simulink model "RoboticFish_NGC"  (R2023b)
settings: Solver=ode4  StartTime=0.0  StopTime=89  FixedStep=0.00025  RelTol=1e-3  EnableMultiTasking=on
undefined symbols (not defined in the file): Ref, uCMD
libraries: sharedutil x11, slpidlib x8, dspsigops x2, matrix_library x1, SignalEditorBlockLib x1, vrlib x1
(part 1 of 3)
settings Model: Creator=Waqas Ali Waqar  LastModifiedBy=Dimau
settings SolverCC: ConcurrentTasks=on  AlgebraicLoopSolver=TrustRegion  AutoInsertRateTranBlk=on  InsertRTBMode=Never (minimum delay)
settings DataIOCC: SaveFormat=StructureWithTime
settings OptimizationCC: BlockReduction=off  OptimizeBlockIOStorage=off  BufferReuse=off  GlobalBufferReuse=off  ExpressionFolding=off  PassReuseOutputArgsThreshold=0  LocalBlockOutputs=off  OptimizeBlockOrder=speed  OptimizeDataStoreBuffers=off  BusAssignmentInplaceUpdate=off
settings DebuggingCC: ParameterTunabilityLossMsg=error  UnconnectedInputMsg=warning  UnconnectedOutputMsg=warning  UnconnectedLineMsg=warning
settings HardwareCC: ProdBitPerPointer=32  ProdBitPerSizeT=32  ProdBitPerPtrDiffT=32  ProdLargestAtomicFloat=None  ProdWordSize=32  ProdLongLongMode=on  ProdHWDeviceType=Generic->32-bit x86 compatible
settings ModelReferenceCC: EnableRefExpFcnMdlSchedulingChecks=on
settings SFSimCC: MATLABDynamicMemAlloc=off  CustomCodeUndefinedFunction=UseInterfaceOnly
settings RTWCC: GenerateReport=on  RTWVerbose=off  LaunchReport=on  RTWCompilerOptimization=on  DLArmComputeVersion=19.05
settings CodeAppCC: ForceParamTrailComments=on  OperatorAnnotations=on
settings GRTTargetCC: TargetLangStandard=C89/C90 (ANSI)

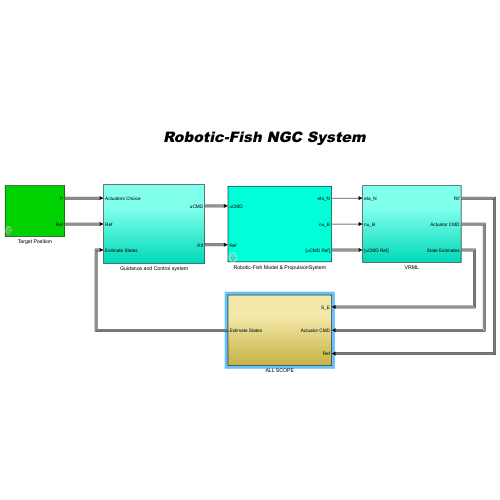
[thumbnail: Simulink's stored preview of the top-level diagram]
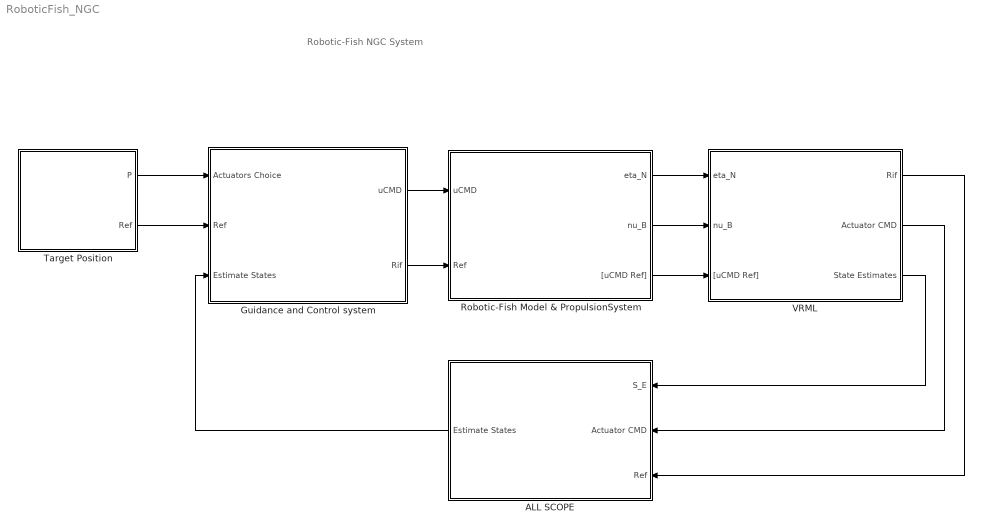
== system RoboticFish_NGC ==
  note: Robotic-Fish NGC System
  ALL SCOPE : Subsystem
  Guidance and Control system : Subsystem
  Robotic-Fish Model & PropulsionSystem : Subsystem  mask{Ig=[0.0198 0 0;0 0.9266 0;0 0 0.9266], m=11.3, rho=1000, R=0.06, L=1, cdf=0.5, cdt=1, W=107.91, B=107.91, rG_B=[0;0;0], rB_B=[0;0;0], DL=diag([0;0;0;0;0;0]), Kt0=1.16, Km1=0.5, Kt1=0.5, Km2=0.073, Kt2=1.26, beta=-4.95, Kl1=0.5, sigma=-3.52, Kl2=5.16, epsilon=-3.51, c=0.1, S=0, a0=0, a2=0, a1=0, Theta0deg=23, cL=2, xfin=0.11, yfin=0.11, zfin=0.75, Max_Delta=45, Min_Delta=-45, Sfin=0.017, HT1Max=1.12, e1=[1;0;0], r1=[0;-0.11;0], HT2Max=1.12, e2=[1;0;0], r2=[0;0.11;0], VT1Max=1.12, e3=[0;0;1], r3=[0;0;-0.03]}
      mask prompts: Ig "Inertia Tensor Ig (Kg*m^2)"; m "Mass m (Kg)"; rho "Seawater Density rho (Kg/m)"; R "Body Radius R (m)"; L "Body Lenght L (m)"; cdf "Drag Weight cdf"; cdt "Drag Weight cdt [0.8-1.2]"; W "Weight (N)"; B "Buoyancy (N)"; rG_B "rG_B (m)"; rB_B "rB_B (m)"; DL "Linear Damping Matrix"; c "c-Foil Mean Chord (m)"; S "S-Foil area (m^2)"; a0 "a0 (Kg*m^2)"; a2 "a2 (Kg*m^2)"; a1 "a1 (Kg*m^2)"; Theta0deg "Theta0-Oscillation amplitude (deg)"; cL "fin lift coefficient  cL"; xfin "fin axial position xfin (m)"; yfin "fin axial position yfin (m)"; zfin "fin axial position zfin (m)"; Max_Delta "Max fin rotation angle (deg)"; Min_Delta "Min fin rotation angle (deg)"; Sfin "fin platform area Sfin (m^2)"; HT1Max "Max Thrust (HT1):"; e1 "e1 (HT1):"; r1 "r1 (HT1):"; HT2Max "Max Thrust (HT2):"; e2 "e2 (HT2 ):"; r2 "r2 (HT2):"; VT1Max "Max Thrust (VT1):"; e3 "e3 (VT1):"; r3 "r3 (VT1):"
      mask init:
      | %%%%%%%%%%%%%%%%%%%%%%%%%%%%%%%%%%%%%%%%%%%%%%%%%%%%%%%
      | %%%%%%%%%%%%%%%%%%%  DINAMICA  %%%%%%%%%%%%%%%%%%%%%%%%
      | %%%%%%%%%%%%%%%%%%%%%%%%%%%%%%%%%%%%%%%%%%%%%%%%%%%%%%%
      | 
      | % Matrice di inerzia del corpo rigido
      | Ib = Ig-m*skewsymm(rG_B)*skewsymm(rG_B);
      | MRB = [m*eye(3,3) -m*skewsymm(rG_B); m*skewsymm(rG_B) Ib];
      | 
      | %Masse aggiunte
      | X_udot = 0.1*m;
      | Y_vdot = pi*rho*R^2*L;
      | Z_wdot = pi*rho*R^2*L;
      | K_pdot = 0;
      | M_qdot = (pi*rho*R^2*L^3)/12;
      | N_rdot = (pi*rho*R^2*L^3)/12;
      | 
      | %Matrice delle masse aggiunte
      | MA = diag([X_udot;Y_vdot;Z_wdot;K_pdot;M_qdot;N_rdot]);
      | 
      | %Matrice di inerzia (incluse le masse aggiunte)
      | M = MRB + MA;
      | inv_M = inv(M);
      | M11 = MA(1:3,1:3);    M12 = MA(1:3,4:6);
      | M21 = MA(4:6,1:3);    M22 = MA(4:6,4:6);
      | 
      | %%Attrito viscoso
      | 
      | %Aree
      | Af = pi*R^2;
      | At = 2*pi*R;
      | 
      | %Coefficienti
      | X_uu = 2*rho*Af*cdf/2;
      | Y_vv = rho*At*cdt/2;
      | Z_ww = rho*At*cdt/2;
      | K_pp = (rho*At*cdt*L^3)/16;
      | M_qq = (rho*At*cdt*L^3)/16;
      | N_rr = (rho*At*cdt*L^3)/16;
      | 
      | dQ = ([X_uu;Y_vv;Z_ww;K_pp;M_qq;N_rr]);
      | 
      | 
      | %%%%%%%%%%%%%%%%%%%%%%%%%%%%%%%%%%%%%%%%%%%%%%%%%%%%%%%
      | %%%%%%%%%%%%%%%%%%%  PROP HT3  %%%%%%%%%%%%%%%%%%%%%%%%
      | %%%%%%%%%%%%%%%%%%%%%%%%%%%%%%%%%%%%%%%%%%%%%%%%%%%%%%%
      | 
      | Theta0=Theta0deg*pi/180
      | TanTheta0=tan(Theta0)
      | 
      | %%%%%%%%%%%%%%%%%%%%%%%%%%%%%%%%%%%%%%%%%%%%%%%%%%%%%%%
      | %%%%%%%%%%%%%%%%%%%  PROP HT1 HT2 VT1  %%%%%%%%%%%%%%%%
      | %%%%%%%%%%%%%%%%%%%%%%%%%%%%%%%%%%%%%%%%%%%%%%%%%%%%%%%
      | 
      | K1 = HT1Max*9.81;
      | K2 = HT2Max*9.81;
      | K3 = VT1Max*9.81;
      | HT_prop = [e1 e2;skewsymm(r1)*e1 skewsymm(r2)*e2]*diag([K1;K2]);
      | VT_prop = [e3 ;skewsymm(r3)*e3 ]*K3;
      | 
      | 
      | %%%%%%%%%%%%%%%%%%%%%%%%%%%%%%%%%%%%%%%%%%%%%%%%%%%%%%%
      | %%%%%%%%%%%%%%%%%%%  PROP VT1 VT2  %%%%%%%%%%%%%%%%%%%%
      | %%%%%%%%%%%%%%%%%%%%%%%%%%%%%%%%%%%%%%%%%%%%%%%%%%%%%%%
      | 
      | Max_Delta_rad=Max_Delta*pi/180;
      | Min_Delta_rad=Min_Delta*pi/180;
      mask DialogControl DescGroupVar Prompt: Robotic Fish Paramteres
      mask DialogControl Container14 Prompt: Robotic Fish Parameters
      mask DialogControl Container17 Prompt: Caudal Fin Parameters
      mask DialogControl Container18 Prompt: Pectoral Fins Parameters
      mask DialogControl Container19 Prompt: Thrusters Parameters
  Target Position : Subsystem  mask{AC=Only Caudal Fin, ST=Way-Points based Path, Xr=10, Yr=0, Zr=0}
      mask init:
      | if (ST == 1)
      |     Flag=0;
      | end
      | if (ST == 2)
      |     Flag=1;
      | end
      | 
      | if (AC == 1)
      |     PropChoice=0;
      | end
      | if (AC == 2)
      |     PropChoice=1;
      | end
      | if (AC == 3)
      |     PropChoice=2;
      | end
      mask TypeOptions AC: Normal | Only Propeller | Only Caudal Fin
      mask TypeOptions ST: Way-Points based Path | Way-Point Position
      mask DialogControl DescGroupVar Prompt: Target Position
      mask DialogControl Container8 Prompt: Actuator Choice
      mask DialogControl Container7 Prompt: Select Target
      mask DialogControl Container9 Prompt: Way-Point position
  "VRML " : Subsystem
  wires:
  Robotic-Fish Model & PropulsionSystem/2(nu_B) -> "VRML "/2(nu_B)
  Target Position/1(" P") -> Guidance and Control system/1(Actuators Choice)
  Robotic-Fish Model & PropulsionSystem/1(eta_N) -> "VRML "/1(eta_N)
  Target Position/2(Ref) -> Guidance and Control system/2(Ref)
  ALL SCOPE/1(Estimate States) -> Guidance and Control system/3("Estimate States ")
  "VRML "/3(State Estimates) -> ALL SCOPE/1(S_E)
  "VRML "/2(Actuator CMD) -> ALL SCOPE/2(Actuator CMD)
  "VRML "/1(Rif) -> ALL SCOPE/3(Ref)
  Robotic-Fish Model & PropulsionSystem/3("[uCMD Ref]") -> "VRML "/3("[uCMD Ref]")
  Guidance and Control system/1(uCMD) -> Robotic-Fish Model & PropulsionSystem/1(uCMD)
  Guidance and Control system/2(Rif) -> Robotic-Fish Model & PropulsionSystem/2(Ref)

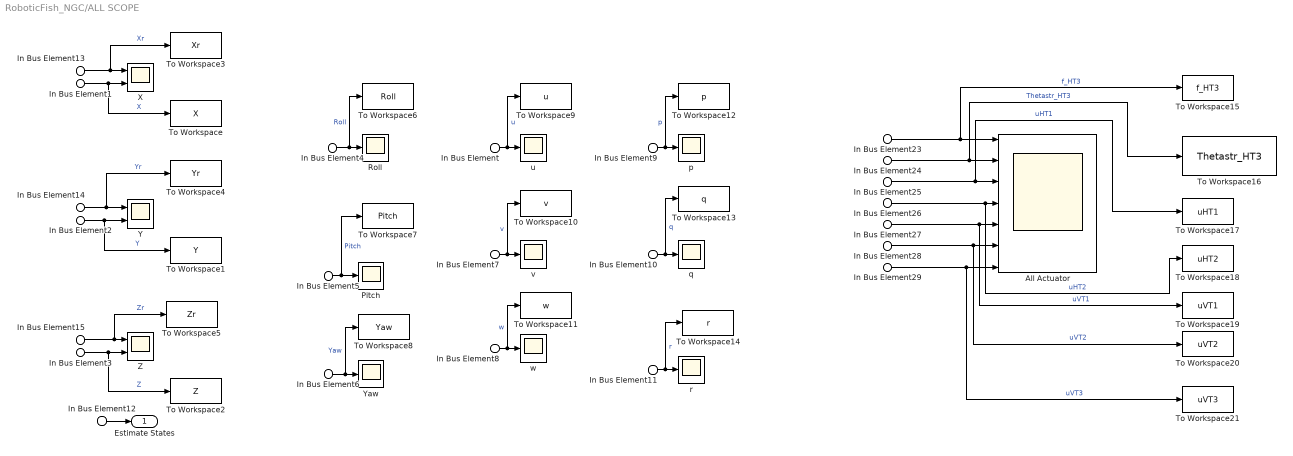
== system RoboticFish_NGC/ALL SCOPE ==
  In Bus Element12 : Inport  PortName=S_E
  In Bus Element2 : Inport  PortName=S_E  Element=Position.Y
  In Bus Element3 : Inport  PortName=S_E  Element=Position.Z
  In Bus Element4 : Inport  PortName=S_E  Element=Position.Roll
  In Bus Element5 : Inport  PortName=S_E  Element=Position.Pitch
  In Bus Element6 : Inport  PortName=S_E  Element=Position.Yaw
  In Bus Element1 : Inport  PortName=S_E  Element=Position.X
  In Bus Element : Inport  PortName=S_E  Element=Velocity.u
  In Bus Element7 : Inport  PortName=S_E  Element=Velocity.v
  In Bus Element8 : Inport  PortName=S_E  Element=Velocity.w
  In Bus Element9 : Inport  PortName=S_E  Element=Velocity.p
  In Bus Element10 : Inport  PortName=S_E  Element=Velocity.q
  In Bus Element11 : Inport  PortName=S_E  Element=Velocity.r
  In Bus Element23 : Inport  Port=2  PortName=Actuator CMD  Element=f_HT3
  In Bus Element24 : Inport  Port=2  PortName=Actuator CMD  Element=Thetastr_HT3
  In Bus Element25 : Inport  Port=2  PortName=Actuator CMD  Element=uHT1
  In Bus Element26 : Inport  Port=2  PortName=Actuator CMD  Element=uHT2
  In Bus Element27 : Inport  Port=2  PortName=Actuator CMD  Element=uVT1
  In Bus Element28 : Inport  Port=2  PortName=Actuator CMD  Element=D_VT2
  In Bus Element29 : Inport  Port=2  PortName=Actuator CMD  Element=D_VT3
  In Bus Element13 : Inport  Port=3  PortName=Ref  Element=Xr
  In Bus Element14 : Inport  Port=3  PortName=Ref  Element=Yr
  In Bus Element15 : Inport  Port=3  PortName=Ref  Element=Zr
  All Actuator : Scope  NumInputPorts=7
  Pitch : Scope
  Roll : Scope
  To Workspace : ToWorkspace  VariableName=X  SampleTime=-1
  To Workspace1 : ToWorkspace  VariableName=Y  SampleTime=-1
  To Workspace10 : ToWorkspace  VariableName=v  SampleTime=-1
  To Workspace11 : ToWorkspace  VariableName=w  SampleTime=-1
  To Workspace12 : ToWorkspace  VariableName=p  SampleTime=-1
  To Workspace13 : ToWorkspace  VariableName=q  SampleTime=-1
  To Workspace14 : ToWorkspace  VariableName=r  SampleTime=-1
  To Workspace15 : ToWorkspace  VariableName=f_HT3  SampleTime=-1
  To Workspace16 : ToWorkspace  VariableName=Thetastr_HT3  SampleTime=-1
  To Workspace17 : ToWorkspace  VariableName=uHT1  SampleTime=-1
  To Workspace18 : ToWorkspace  VariableName=uHT2  SampleTime=-1
  To Workspace19 : ToWorkspace  VariableName=uVT1  SampleTime=-1
  To Workspace2 : ToWorkspace  VariableName=Z  SampleTime=-1
  To Workspace20 : ToWorkspace  VariableName=uVT2  SampleTime=-1
  To Workspace21 : ToWorkspace  VariableName=uVT3  SampleTime=-1
  To Workspace3 : ToWorkspace  VariableName=Xr  SampleTime=-1
  To Workspace4 : ToWorkspace  VariableName=Yr  SampleTime=-1
  To Workspace5 : ToWorkspace  VariableName=Zr  SampleTime=-1
  To Workspace6 : ToWorkspace  VariableName=Roll  SampleTime=-1
  To Workspace7 : ToWorkspace  VariableName=Pitch  SampleTime=-1
  To Workspace8 : ToWorkspace  VariableName=Yaw  SampleTime=-1
  To Workspace9 : ToWorkspace  VariableName=u  SampleTime=-1
  X : Scope  NumInputPorts=2
  Y : Scope  NumInputPorts=2
  Yaw : Scope
  Z : Scope  NumInputPorts=2
  p : Scope
  q : Scope
  r : Scope
  u : Scope
  v : Scope
  w : Scope
  Estimate States : Outport  VectorParamsAs1DForOutWhenUnconnected=off
  wires:
  In Bus Element4/1 -> To Workspace6/1, Roll/1  "Roll"
  In Bus Element5/1 -> To Workspace7/1, Pitch/1  "Pitch"
  In Bus Element6/1 -> To Workspace8/1, Yaw/1  "Yaw"
  In Bus Element/1 -> To Workspace9/1, u/1  "u"
  In Bus Element7/1 -> To Workspace10/1, v/1  "v"
  In Bus Element8/1 -> To Workspace11/1, w/1  "w"
  In Bus Element9/1 -> To Workspace12/1, p/1  "p"
  In Bus Element10/1 -> To Workspace13/1, q/1  "q"
  In Bus Element11/1 -> To Workspace14/1, r/1  "r"
  In Bus Element12/1 -> Estimate States/1
  In Bus Element15/1 -> To Workspace5/1, Z/1  "Zr"
  In Bus Element3/1 -> To Workspace2/1, Z/2  "Z"
  In Bus Element2/1 -> Y/2, To Workspace1/1  "Y"
  In Bus Element14/1 -> To Workspace4/1, Y/1  "Yr"
  In Bus Element23/1 -> To Workspace15/1, All Actuator/1  "f_HT3"
  In Bus Element24/1 -> All Actuator/2, To Workspace16/1  "Thetastr_HT3"
  In Bus Element25/1 -> To Workspace17/1, All Actuator/3  "uHT1"
  In Bus Element26/1 -> To Workspace18/1, All Actuator/4  "uHT2"
  In Bus Element27/1 -> All Actuator/5, To Workspace19/1  "uVT1"
  In Bus Element28/1 -> All Actuator/6, To Workspace20/1  "uVT2"
  In Bus Element29/1 -> All Actuator/7, To Workspace21/1  "uVT3"
  In Bus Element1/1 -> X/2, To Workspace/1  "X"
  In Bus Element13/1 -> X/1, To Workspace3/1  "Xr"

== system RoboticFish_NGC/Guidance and Control system ==
  note: [X Y Z]
  note: [X Y Z] at the
      | current time
  note: [D, Yaw_d, Ze]
  note: "uCMD" vector is formed by the control signals of the robotic fish actuators
  note: Waypoints [Xr Yr Zr]
  Actuators Choice : Inport
  Ref : Inport  Port=2
  "Estimate States " : Inport  Port=3
  " Control system" : Subsystem
  " Guidance system" : Subsystem
  uCMD : Outport  VectorParamsAs1DForOutWhenUnconnected=off
  Rif : Outport  Port=2  VectorParamsAs1DForOutWhenUnconnected=off
  wires:
  "Estimate States "/1 -> " Guidance system"/2(Estimate States I)
  Ref/1 -> Rif/1, " Guidance system"/1(Ref)
  " Guidance system"/1("LOS ") -> " Control system"/1(LOS)
  Actuators Choice/1 -> " Control system"/2(Actuators Choice)
  " Guidance system"/2(Estimate States O) -> " Control system"/3(Estimate States)
  " Control system"/1(uCMD) -> uCMD/1

== system RoboticFish_NGC/Robotic-Fish Model & PropulsionSystem ==
  uCMD : Inport
  In Bus Element1 : Inport  Port=2  PortName=Ref
  Bus Creator : BusCreator  Inputs=2
  Memory : Memory
  Propulsion System : Subsystem
  RF Dynamics and Kinematics (Attitude rappresentation: Quaternions) : Subsystem
      mask Display: image('RF.png');
  eta_N : Outport  VectorParamsAs1DForOutWhenUnconnected=off
  nu_B : Outport  Port=2  VectorParamsAs1DForOutWhenUnconnected=off
  "[uCMD Ref]" : Outport  Port=3  VectorParamsAs1DForOutWhenUnconnected=off
  wires:
  RF Dynamics and Kinematics (Attitude rappresentation: Quaternions)/1(nu_B) -> nu_B/1, Memory/1  "[u    v    w    p    q    r]"
  Memory/1 -> Propulsion System/1(nu_B)
  RF Dynamics and Kinematics (Attitude rappresentation: Quaternions)/2(eta_N) -> eta_N/1  "[x   y   z  q0  q1  q2  q3]"
  uCMD/1 -> Propulsion System/2(uCMD)
  Propulsion System/2(ucmd) -> Bus Creator/1  "uCMD"
  Propulsion System/1(Tau_B) -> RF Dynamics and Kinematics (Attitude rappresentation: Quaternions)/1(tau_B)  "[Tau_X, Tau_Y, Tau_Z, Tau_Roll, Tau_Pitch, Tau_Yaw]"
  In Bus Element1/1 -> Bus Creator/2  "Ref"
  Bus Creator/1 -> "[uCMD Ref]"/1

== system RoboticFish_NGC/Target Position ==
  note: By means of a radio button, it is possible to choose how the vehicle is actuated.
      |
      | 0) “Normal” operation which involves the use of the caudal fin for surge motion, the lateral propellers for steering.
      |
      | 1) “Only Propeller” operation, where the propellers are used for both surge motion and steering.
      |
      | 2) "Only Caudal Fin" operation which involves only the use of the caudal fin for surge motion and steering.
  note: The control panel provides a radio button that allows you to choose the type of target to be reached.
      |
      | 0) “Way-Points based Path” allows you to choose Path consisting of a multiple waypoint that can be generated from the “Waypoints generator” block, which is a Simulink block that creates a group of signals (“Signal Builder”).
      |
      | 1) “Way-Point Position” consists in choosing the x y z coordinate of the reference, essentially it consists of a set-point.
  note: u1 (if u2 = 1)
  note: u3 (if u2 = 0)
  note: Waypoints [Xr Yr Zr]
  note: u2
  note: u3 Waypoints based Path
  note: u1 Waypoint Position
  Bus Creator : BusCreator  Inputs=3
  Bus Creator1 : BusCreator  Inputs=3
  Constant : Constant  Value=Flag
  Constant1 : Constant  Value=Xr
  Constant2 : Constant  Value=Yr
  Constant3 : Constant  Value=Zr
  Constant4 : Constant  Value=PropChoice
  Signal Editor : SignalEditorBlockLib/Signal Editor  FileName=waypoint_generator.mat  ActiveScenario=Scenario  ActiveSignal=Xr  IsBus=off  OutputBusObjectStr=Bus: BusObject  SampleTime=0  Interpolate=off  ZeroCross=off  OutputAfterFinalValue=Setting to zero  Unit=inherit  PreserveSignalName=on  ApplySigPropsToAllScenarios=on  ApplySigPropsToAllSignals=on
  Switch : Switch  Criteria=u2 > Threshold  SaturateOnIntegerOverflow=off  InputSameDT=off
  Bus Element Out : Outport  VectorParamsAs1DForOutWhenUnconnected=off  PortName=P  Element=Actuators Choice
  Ref : Outport  Port=2  VectorParamsAs1DForOutWhenUnconnected=off
  wires:
  Constant/1 -> Switch/2
  Bus Creator1/1 -> Switch/3
  Bus Creator/1 -> Switch/1
  Switch/1 -> Ref/1
  Constant3/1 -> Bus Creator/3  "Zr"
  Constant2/1 -> Bus Creator/2  "Yr"
  Constant1/1 -> Bus Creator/1  "Xr"
  Constant4/1 -> Bus Element Out/1  "PCHOICE"
  Signal Editor/1 -> Bus Creator1/1
  Signal Editor/2 -> Bus Creator1/2
  Signal Editor/3 -> Bus Creator1/3

== system RoboticFish_NGC/VRML  ==
  eta_N : Inport
  nu_B : Inport  Port=2
  In Bus Element1 : Inport  Port=3  PortName=[uCMD Ref]  Element=uCMD
  In Bus Element : Inport  Port=3  PortName=[uCMD Ref]  Element=Ref
  In Bus Element2 : Inport  Port=3  PortName=[uCMD Ref]  Element=Ref
  Bus Selector : BusSelector  OutputSignals=uVT3,uVT2,uHT3,uVT1,uHT2,uHT1
  Estimate States : Subsystem
  RF Position and Rotation to VR Translation and Rotation : Subsystem
  RF Virtual Reality Display : vrlib/VR Sink  InstantiateOnLoad=on  SampleTime=0.1  ViewEnable=on  RemoteChange=off  RemoteView=off  FieldsWritten=WayPoint.rotation.4.1.1.double#WayPoint.translation.3.1.1.double#RF.rotation.4.1.1.double#RF.translation.3.1.1.double#VT3.rotation.4.1.1.double#Vt2.rotation.4.1.1.double#HT3.rotation.4.1.1.double#VT1.rotation.4.1.1.double#HT2.rotation.4.1.1.double#HT1.rotation.4.1.1.double#ViewPoints.translation.3.1.1.double  WorldFileName=Final_RF.wrl  AutoView=on  VideoDimensions=[]  AllowVariableSize=off  FigureProperties="{'Position', 'Name', 'Viewpoint', 'CameraBound', 'CameraDirection', 'CameraPosition', 'CameraUpVector', 'ZoomFactor', 'Antialiasing', 'Headlight', 'Lighting', 'NavPanel', 'Sound', 'StatusBar', 'Stereo3D', 'Stereo3DCameraOffset', 'Stereo3DHIT', 'ToolBar', 'Textures', 'Transparency', 'Triad', 'Wireframe', 'NavZones', 'NavMode', 'NavSpeed', 'CaptureFileFormat', 'CaptureFileName', 'Record2DCompressMethod', 'Record2DCompressQuality', 'Record2D', 'Record2DFileName', 'Record2DFPS'; [1.0000000000000000e+00   7.6000000000000000e+01   1.9200000000000000e+03   9.1300000000000000e+02], '', 'RF_UP_CAMERA', 'on', [0.0000000000000000e+00   0.0000000000000000e+00  -1.0000000000000000e+00], [0.0000000000000000e+00   0.0000000000000000e+00   1.8000000000000000e+01], [0.0000000000000000e+00   1.0000000000000000e+00   0.0000000000000000e+00], [1.0000000000000000e+00], 'on', 'on', 'on', 'halfbar', 'on', 'on', 'off', [1.0000000149011612e-01], [0.0000000000000000e+00], 'on', 'on', 'on', 'none', 'off', 'off', 'fly', 'normal', 'tif', '%f_anim_%n.tif', 'auto', [7.5000000000000000e+01], 'off', '%f_anim_%n.avi', 'auto'}"
  Thruster rotation : Subsystem
  WayPoint Position and Rotation To VR Translation and Rotation : Subsystem
  Rif : Outport  VectorParamsAs1DForOutWhenUnconnected=off
  Actuator CMD : Outport  Port=2  VectorParamsAs1DForOutWhenUnconnected=off
  State Estimates : Outport  Port=3  VectorParamsAs1DForOutWhenUnconnected=off
  wires:
  eta_N/1 -> Estimate States/2(eta), RF Position and Rotation to VR Translation and Rotation/1(eta_N)
  nu_B/1 -> Estimate States/1(nu)
  RF Position and Rotation to VR Translation and Rotation/1(VR Rotation) -> WayPoint Position and Rotation To VR Translation and Rotation/2(RF VR Rotation), RF Virtual Reality Display/3
  Estimate States/1(Estimate States) -> State Estimates/1
  In Bus Element2/1 -> WayPoint Position and Rotation To VR Translation and Rotation/1(Waypoint Position)
  Thruster rotation/1(T_rotation) -> Bus Selector/1
  In Bus Element1/1 -> Actuator CMD/1, Thruster rotation/1(uCMD)
  In Bus Element/1 -> Rif/1
  WayPoint Position and Rotation To VR Translation and Rotation/2(Waypoint VR Translation) -> RF Virtual Reality Display/2
  WayPoint Position and Rotation To VR Translation and Rotation/1(Waypoint VR Rotation) -> RF Virtual Reality Display/1
  Bus Selector/1 -> RF Virtual Reality Display/5  "<uVT3>"
  Bus Selector/2 -> RF Virtual Reality Display/6  "<uVT2>"
  Bus Selector/3 -> RF Virtual Reality Display/7  "<uHT3>"
  Bus Selector/4 -> RF Virtual Reality Display/8  "<uVT1>"
  Bus Selector/5 -> RF Virtual Reality Display/9  "<uHT2>"
  Bus Selector/6 -> RF Virtual Reality Display/10  "<uHT1>"
  RF Position and Rotation to VR Translation and Rotation/2(VR Translation) -> RF Virtual Reality Display/11, RF Virtual Reality Display/4

== system RoboticFish_NGC/Guidance and Control system/ Control system ==
  note: [TX TN TZ]
  note: [D, Yaw_d, Ze]
  note: [X Y Z]
  LOS : Inport
  Actuators Choice : Inport  Port=2
  Estimate States : Inport  Port=3
  Control Allocator : Subsystem
  Control Law : Subsystem
  uCMD : Outport  VectorParamsAs1DForOutWhenUnconnected=off
  wires:
  LOS/1 -> Control Law/1(LOS)
  Control Allocator/1(uCMD) -> uCMD/1
  Actuators Choice/1 -> Control Law/2(P)
  Control Law/1(Tin) -> Control Allocator/1(Tin)
  Control Law/2(Actuators Choice O) -> Control Allocator/2(Actuators Choice)
  Estimate States/1 -> Control Law/3(Estimate States)

== system RoboticFish_NGC/Guidance and Control system/ Guidance system ==
  note: As output it returns the vector “LOS” composed of the distance D, calculated by the "Distance" block, the yaw angle Yaw_d, calculated by the "LOS law" block and the difference between Zr and Z, that is Ze. Furthermore, it returns as second output the “Estimate States” vector.
  note: [D, Yaw_d, Ze]
  note: This block takes as input the “ref” vector consisting of Xr Yr and Zr and as a second input the vector “Estimate States” containing the position, the orientation, the linear and angular velocities of the robot at the current time, by selecting only the x y z coordinates of the current position of the vehicle [X Y Z].
  In Bus Element9 : Inport  PortName=Ref  Element=Xr
  In Bus Element10 : Inport  PortName=Ref  Element=Yr
  In Bus Element8 : Inport  PortName=Ref  Element=Zr
  In Bus Element3 : Inport  Port=2  PortName=Estimate States I
  In Bus Element4 : Inport  Port=2  PortName=Estimate States I  Element=Position.X
  In Bus Element5 : Inport  Port=2  PortName=Estimate States I  Element=Position.Y
  In Bus Element6 : Inport  Port=2  PortName=Estimate States I  Element=Position.Z
  Bus Creator : BusCreator  Inputs=3
  Distance : Subsystem
  LOS law : Subsystem
  Mux1 : Mux  Inputs=3
  Mux4 : Mux  Inputs=3
  Selector : Selector  InputPortWidth=3  IndexOptions=Index vector (dialog)  Indices=[3]  OutputSizes=1
  Selector1 : Selector  InputPortWidth=3  IndexOptions=Index vector (dialog)  Indices=[1 2]  OutputSizes=1
  Selector2 : Selector  InputPortWidth=3  IndexOptions=Index vector (dialog)  Indices=[1 2]  OutputSizes=1
  Sum2 : Sum  Inputs=|+-
  "LOS " : Outport  VectorParamsAs1DForOutWhenUnconnected=off
  Estimate States O : Outport  Port=2  VectorParamsAs1DForOutWhenUnconnected=off
  wires:
  In Bus Element3/1 -> Estimate States O/1
  In Bus Element4/1 -> Mux1/1
  In Bus Element5/1 -> Mux1/2
  LOS law/1(Yaw_d) -> Bus Creator/2  "Yaw_d"
  Selector/1 -> Bus Creator/3  "Ze"
  Bus Creator/1 -> "LOS "/1
  Sum2/1 -> Selector1/1, Selector/1, Selector2/1  "[Xe Ye Ze]"
  Distance/1(D) -> Bus Creator/1  "D"
  In Bus Element9/1 -> Mux4/1
  In Bus Element10/1 -> Mux4/2
  Mux4/1 -> Sum2/1  "[Xr Yr Zr]"
  Mux1/1 -> Sum2/2  "[X Y Z]"
  Selector1/1 -> Distance/1("[Xe Ye]")  "[Xe Ye]"
  Selector2/1 -> LOS law/1("[Xe Ye]")  "[Xe Ye]"
  In Bus Element6/1 -> Mux1/3
  In Bus Element8/1 -> Mux4/3

== system RoboticFish_NGC/Robotic-Fish Model & PropulsionSystem/Propulsion System ==
  nu_B : Inport
  In Bus Element : Inport  Port=2  PortName=uCMD
  In Bus Element1 : Inport  Port=2  PortName=uCMD  Element=f_HT3
  In Bus Element4 : Inport  Port=2  PortName=uCMD  Element=uHT2
  In Bus Element5 : Inport  Port=2  PortName=uCMD  Element=uVT1
  In Bus Element6 : Inport  Port=2  PortName=uCMD  Element=uVT2
  In Bus Element7 : Inport  Port=2  PortName=uCMD  Element=uVT3
  In Bus Element8 : Inport  Port=2  PortName=uCMD  Element=Thetastr_HT3
  In Bus Element2 : Inport  Port=2  PortName=uCMD  Element=uHT1
  Bus Creator : BusCreator  Inputs=2
  Bus Creator1 : BusCreator  Inputs=2
  Horizontal Force and Moment (Tau_H) : Subsystem
  Subsystem : Subsystem
  Sum : Sum  Inputs=|++
  Vertical Force and Moment (Tau_V) : Subsystem
  Tau_B : Outport  VectorParamsAs1DForOutWhenUnconnected=off
  ucmd : Outport  Port=2  VectorParamsAs1DForOutWhenUnconnected=off
  wires:
  nu_B/1 -> Horizontal Force and Moment (Tau_H)/4(nu_B), Vertical Force and Moment (Tau_V)/1(nu_B)
  Sum/1 -> Tau_B/1  "Horizontal_Tau+Vertical_Tau"
  Horizontal Force and Moment (Tau_H)/1(Horizontal _Tau) -> Sum/1
  Vertical Force and Moment (Tau_V)/1(Vertical_Tau) -> Sum/2
  In Bus Element6/1 -> Bus Creator/1
  In Bus Element7/1 -> Bus Creator/2
  Bus Creator/1 -> Vertical Force and Moment (Tau_V)/3("[uVT2 uVT3]")
  In Bus Element5/1 -> Vertical Force and Moment (Tau_V)/2(uVT1)
  In Bus Element4/1 -> Horizontal Force and Moment (Tau_H)/3(uHT2)
  In Bus Element2/1 -> Horizontal Force and Moment (Tau_H)/2(uHT1)
  In Bus Element1/1 -> Bus Creator1/1
  In Bus Element8/1 -> Bus Creator1/2
  Bus Creator1/1 -> Horizontal Force and Moment (Tau_H)/1(uHT3)
  Vertical Force and Moment (Tau_V)/2("[Delta_VT2 Delta_VT3]") -> Subsystem/1(D_uVT2  D_uVT3)
  In Bus Element/1 -> Subsystem/2(uCMD)
  Subsystem/1("ucmd ") -> ucmd/1

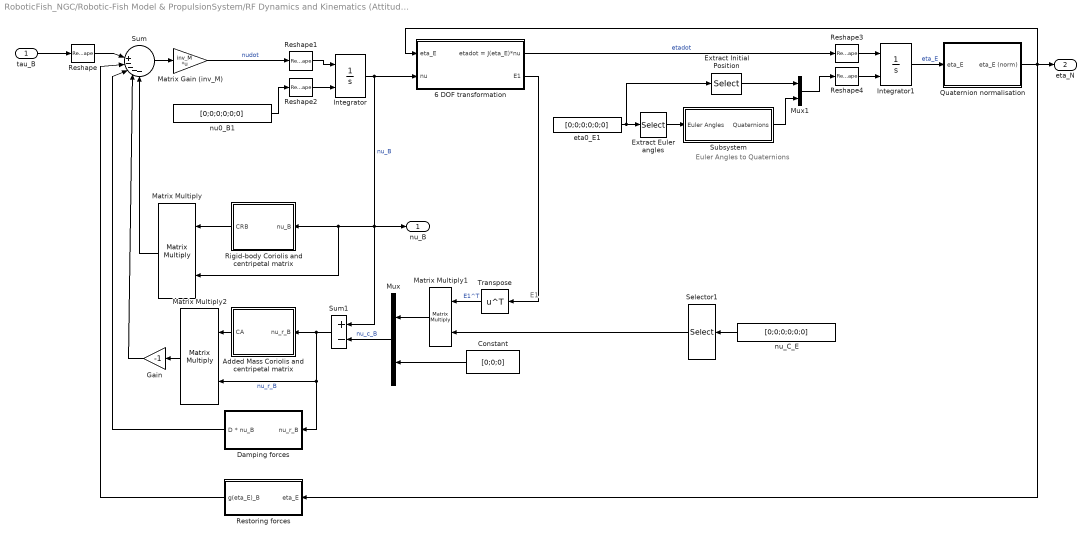
== system RoboticFish_NGC/Robotic-Fish Model & PropulsionSystem/RF Dynamics and Kinematics (Attitude rappresentation: Quaternions) ==
  note: E1
  note: Euler Angles to Quaternions
  tau_B : Inport
  6 DOF transformation : Subsystem  AncestorBlock=MarineGNC/Library blocks/Axes transformations/6 DOF transformation
  Added Mass Coriolis and centripetal matrix : Subsystem
  Constant : Constant  Value=[0;0;0]
  Damping forces : Subsystem
  Extract Euler angles : Selector  InputPortWidth=6  IndexOptions=Index vector (dialog)  Indices=[4 5 6]  OutputSizes=1
  Extract Initial Position : Selector  InputPortWidth=6  IndexOptions=Index vector (dialog)  Indices=[1 2 3]  OutputSizes=1
  Gain : Gain  Gain=-1
  Integrator : Integrator  InitialConditionSource=external
  Integrator1 : Integrator  InitialConditionSource=external
  Matrix Gain (inv_M) : Gain  Gain=inv_M  Multiplication=Matrix(K*u)  SaturateOnIntegerOverflow=on  OutDataTypeStr=Inherit: Same as input  ParamDataTypeStr=Inherit: Same as input
  Matrix Multiply : Product  Multiplication=Matrix(*)
  Matrix Multiply1 : Product  Multiplication=Matrix(*)
  Matrix Multiply2 : Product  Multiplication=Matrix(*)
  Mux : Mux  Inputs=2
  Mux1 : Mux  Inputs=2
  Quaternion normalisation : Subsystem
  Reshape{,1..4} (5 alike) : Reshape  OutputDimensionality=Column vector (2-D)
  Restoring forces : Subsystem
  Rigid-body Coriolis and centripetal matrix : Subsystem
  Selector1 : Selector  InputPortWidth=6  IndexOptions=Index vector (dialog)  Indices=[1 2 3]  OutputSizes=1
  Subsystem : Subsystem
  Sum : Sum  Inputs=|||+----  SaturateOnIntegerOverflow=on
  Sum1 : Sum  Inputs=+-
  Transpose : Math  Operator=transpose  SignedPower=on
  eta0_E1 : Constant  Value=[0;0;0;0;0;0]
  nu0_B1 : Constant  Value=[0;0;0;0;0;0]
  nu_C_E : Constant  Value=[0;0;0;0;0;0]
  nu_B : Outport  VectorParamsAs1DForOutWhenUnconnected=off
  eta_N : Outport  Port=2  VectorParamsAs1DForOutWhenUnconnected=off
  wires:
  Subsystem/1(Quaternions) -> Mux1/2
  Restoring forces/1(g(eta_E)_B) -> Sum/2
  eta0_E1/1 -> Extract Euler angles/1, Extract Initial Position/1
  Extract Initial Position/1 -> Mux1/1
  Selector1/1 -> Matrix Multiply1/2
  Matrix Gain (inv_M)/1 -> Reshape1/1  "nudot"
  Reshape4/1 -> Integrator1/2
  tau_B/1 -> Reshape/1
  Constant/1 -> Mux/2
  Quaternion normalisation/1(eta_E (norm)) -> 6 DOF transformation/1(eta_E), eta_N/1, Restoring forces/1(eta_E)
  Mux1/1 -> Reshape4/1
  nu_C_E/1 -> Selector1/1
  Extract Euler angles/1 -> Subsystem/1("Euler Angles ")
  Reshape/1 -> Sum/1
  Reshape1/1 -> Integrator/1
  Damping forces/1(D * nu_B) -> Sum/3
  Integrator1/1 -> Quaternion normalisation/1(eta_E)  "eta_E"
  6 DOF transformation/2(E1) -> Transpose/1
  Sum/1 -> Matrix Gain (inv_M)/1
  Rigid-body Coriolis and centripetal matrix/1(CRB) -> Matrix Multiply/1
  Mux/1 -> Sum1/2  "nu_c_B"
  6 DOF transformation/1(etadot = J(eta_E)*nu) -> Reshape3/1  "etadot"
  Integrator/1 -> 6 DOF transformation/2(nu), nu_B/1, Sum1/1, Rigid-body Coriolis and centripetal matrix/1(nu_B), Matrix Multiply/2  "nu_B"
  Matrix Multiply/1 -> Sum/5
  Transpose/1 -> Matrix Multiply1/1  "E1^T"
  Matrix Multiply1/1 -> Mux/1
  Sum1/1 -> Damping forces/1(nu_r_B), Matrix Multiply2/2, Added Mass Coriolis and centripetal matrix/1(nu_r_B)  "nu_r_B"
  nu0_B1/1 -> Reshape2/1
  Added Mass Coriolis and centripetal matrix/1(CA) -> Matrix Multiply2/1
  Reshape2/1 -> Integrator/2
  Reshape3/1 -> Integrator1/1
  Matrix Multiply2/1 -> Gain/1
  Gain/1 -> Sum/4

== system RoboticFish_NGC/VRML /Estimate States ==
  nu : Inport
  eta : Inport  Port=2
  Gain : Gain  Gain=180/pi
  Mux : Mux  Inputs=2
  Quaternions to Euler Angles : Subsystem
  Subsystem : Subsystem
  eta1_E=[x,y,z]1 : Selector  InputPortWidth=7  IndexOptions=Index vector (dialog)  Indices=[1 2 3]  OutputSizes=1
  eta2_E=[q0,q1,q2,q3] : Selector  InputPortWidth=7  IndexOptions=Index vector (dialog)  Indices=[4 5 6 7]  OutputSizes=1
  Estimate States : Outport  VectorParamsAs1DForOutWhenUnconnected=off
  wires:
  eta2_E=[q0,q1,q2,q3]/1 -> Quaternions to Euler Angles/1(Quaternions)
  Mux/1 -> Subsystem/1(Position)
  eta1_E=[x,y,z]1/1 -> Mux/1
  eta/1 -> eta2_E=[q0,q1,q2,q3]/1, eta1_E=[x,y,z]1/1
  Subsystem/1(State Estimate) -> Estimate States/1
  Quaternions to Euler Angles/1(Euler Angles) -> Gain/1
  nu/1 -> Subsystem/2(nu_B)
  Gain/1 -> Mux/2

== system RoboticFish_NGC/VRML /RF Position and Rotation to VR Translation and Rotation ==
  eta_N : Inport
  Orientation to VR Rotation : Subsystem
  Position to VR Translation : Subsystem
  eta1_N=[x,y,z] : Selector  InputPortWidth=7  IndexOptions=Index vector (dialog)  Indices=[1 2 3]  OutputSizes=1
  eta2_N=[q0,q1,q2,q3] : Selector  InputPortWidth=7  IndexOptions=Index vector (dialog)  Indices=[4 5 6 7]  OutputSizes=1
  VR Rotation : Outport  VectorParamsAs1DForOutWhenUnconnected=off
  VR Translation : Outport  Port=2  VectorParamsAs1DForOutWhenUnconnected=off
  wires:
  eta2_N=[q0,q1,q2,q3]/1 -> Orientation to VR Rotation/1(Orientation)
  eta1_N=[x,y,z]/1 -> Position to VR Translation/1(Position)
  eta_N/1 -> eta1_N=[x,y,z]/1, eta2_N=[q0,q1,q2,q3]/1
  Orientation to VR Rotation/1(VR Rotation) -> VR Rotation/1
  Position to VR Translation/1(VR Translation) -> VR Translation/1

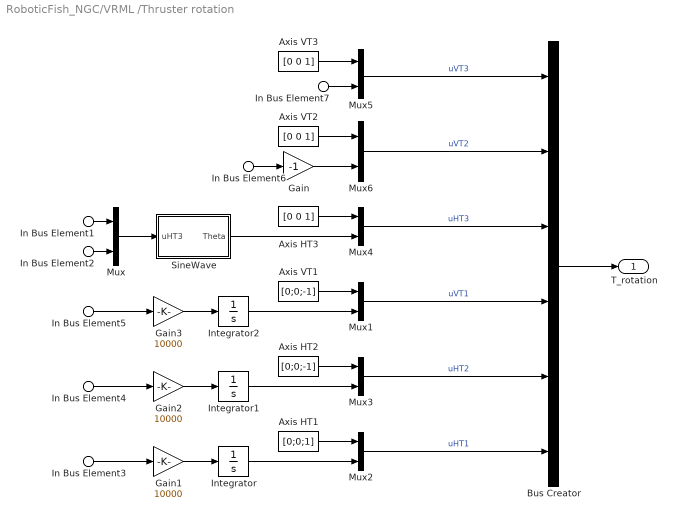
== system RoboticFish_NGC/VRML /Thruster rotation ==
  In Bus Element1 : Inport  PortName=uCMD  Element=f_HT3
  In Bus Element2 : Inport  PortName=uCMD  Element=Thetastr_HT3
  In Bus Element3 : Inport  PortName=uCMD  Element=uHT1
  In Bus Element4 : Inport  PortName=uCMD  Element=uHT2
  In Bus Element5 : Inport  PortName=uCMD  Element=uVT1
  In Bus Element6 : Inport  PortName=uCMD  Element=D_VT2
  In Bus Element7 : Inport  PortName=uCMD  Element=D_VT3
  Axis HT1 : Constant  Value=[0;0;1]
  Axis HT2 : Constant  Value=[0;0;-1]
  Axis HT3 : Constant  Value=[0 0 1]
  Axis VT1 : Constant  Value=[0;0;-1]
  Axis VT2 : Constant  Value=[0 0 1]
  Axis VT3 : Constant  Value=[0 0 1]
  Bus Creator : BusCreator  Inputs=6
  Gain : Gain  Gain=-1
  Gain1 : Gain  Gain=10000
  Gain2 : Gain  Gain=10000
  Gain3 : Gain  Gain=10000
  Integrator : Integrator
  Integrator1 : Integrator
  Integrator2 : Integrator
  Mux{,1..6} (7 alike) : Mux  Inputs=2
  SineWave : Subsystem  mask{Theta0=23}
      mask prompts: Theta0 "Theta0(Degrees)"
      mask init:
      | radTheta0=Theta0*pi/180
  T_rotation : Outport  VectorParamsAs1DForOutWhenUnconnected=off
  wires:
  Gain1/1 -> Integrator/1
  Axis HT3/1 -> Mux4/1
  Integrator1/1 -> Mux3/2
  Axis HT2/1 -> Mux3/1
  Integrator/1 -> Mux2/2
  SineWave/1(Theta) -> Mux4/2
  Integrator2/1 -> Mux1/2
  Axis VT1/1 -> Mux1/1
  Axis VT3/1 -> Mux5/1
  Axis VT2/1 -> Mux6/1
  Gain/1 -> Mux6/2
  Mux5/1 -> Bus Creator/1  "uVT3"
  Mux6/1 -> Bus Creator/2  "uVT2"
  Mux4/1 -> Bus Creator/3  "uHT3"
  Mux1/1 -> Bus Creator/4  "uVT1"
  Mux3/1 -> Bus Creator/5  "uHT2"
  Mux2/1 -> Bus Creator/6  "uHT1"
  Bus Creator/1 -> T_rotation/1
  In Bus Element7/1 -> Mux5/2
  In Bus Element6/1 -> Gain/1
  In Bus Element1/1 -> Mux/1
  In Bus Element2/1 -> Mux/2
  Mux/1 -> SineWave/1(uHT3)
  In Bus Element3/1 -> Gain1/1
  Gain2/1 -> Integrator1/1
  In Bus Element4/1 -> Gain2/1
  In Bus Element5/1 -> Gain3/1
  Gain3/1 -> Integrator2/1
  Axis HT1/1 -> Mux2/1

== system RoboticFish_NGC/VRML /WayPoint Position and Rotation To VR Translation and Rotation ==
  Waypoint Position : Inport
  RF VR Rotation : Inport  Port=2
  Way point Position to VR Translation : Subsystem
  Waypoint VR Rotation : Outport  VectorParamsAs1DForOutWhenUnconnected=off
  Waypoint VR Translation : Outport  Port=2  VectorParamsAs1DForOutWhenUnconnected=off
  wires:
  Way point Position to VR Translation/1(VR Translation) -> Waypoint VR Translation/1
  Waypoint Position/1 -> Way point Position to VR Translation/1(Position)
  RF VR Rotation/1 -> Waypoint VR Rotation/1

== system RoboticFish_NGC/Guidance and Control system/ Control system/Control Allocator ==
  Tin : Inport
  Actuators Choice : Inport  Port=2
  Matrix Multiply : Product  Multiplication=Matrix(*)
  Pseudoinverse choice : Subsystem
  Saturation limits : Subsystem
  uCMD : Outport  VectorParamsAs1DForOutWhenUnconnected=off
  wires:
  Saturation limits/1(uCMD) -> uCMD/1  "f_HT3 Thetastr_HT3  uHT1  uHT2  uVT1  uVT2  uVT3"
  Pseudoinverse choice/1(Pseudoinverse) -> Matrix Multiply/1
  Tin/1 -> Matrix Multiply/2, Pseudoinverse choice/1(Tin)  "[TX TN TZ]"
  Matrix Multiply/1 -> Saturation limits/1(InBus)  "f_HT3 Thetastr_HT3  uHT1  uHT2  uVT2  uVT3  uVT1"
  Actuators Choice/1 -> Pseudoinverse choice/2(Actuators Choice)
